simulink model "Earth_Pointing"  (R2020b)
settings: Solver=ode45  StartTime=0.0  StopTime=5829  RelTol=1e-5
values from neighbouring files (symbols this model uses):
  A = zeros(N_body+N_SP,1)    [main_detumbling.m]    (also in main_earthpointing.m; main_nocontrol.m)
  d = zeros(N_body+N_SP,3)    [main_detumbling.m]    (also in main_earthpointing.m; main_nocontrol.m)
  d_cg = [0.017 0 0]'    [main_detumbling.m]    (also in main_earthpointing.m; main_nocontrol.m)
  I = [Ix Iy Iz]    [main_detumbling.m]    (also in main_earthpointing.m; main_nocontrol.m)
  i = deg2rad(20)    [main_detumbling.m]    (also in main_earthpointing.m; main_nocontrol.m)
  IGRF_coefficients = [1 1 2 2 2 3 3 3 3 4 4 4 ... (832 elements, 104x8)]    [IGRF_coefficients.mat]
  kep = [a; e; i; OM; om; theta]    [main_detumbling.m]    (also in main_earthpointing.m; main_nocontrol.m)
  N = zeros(N_body+N_SP,3)    [main_detumbling.m]    (also in main_earthpointing.m; main_nocontrol.m)
  theta = 0    [PlotEarth.m]    (also in main_detumbling.m = deg2rad(0); main_earthpointing.m = deg2rad(0); main_nocontrol.m = deg2rad(0))
  w_0 = deg2rad([8 13 4])    [main_detumbling.m]    (also in main_earthpointing.m = deg2rad([0 0 0]); main_nocontrol.m)
undefined symbols (not defined in the file or in its folder): deg, IAU, s
libraries: aerolibtransform2 x1, aerolibconvert2 x1, dspmtrx3 x1
settings Model: SimulationMode=accelerator  Creator=GianMarco  LastModifiedBy=GianMarco

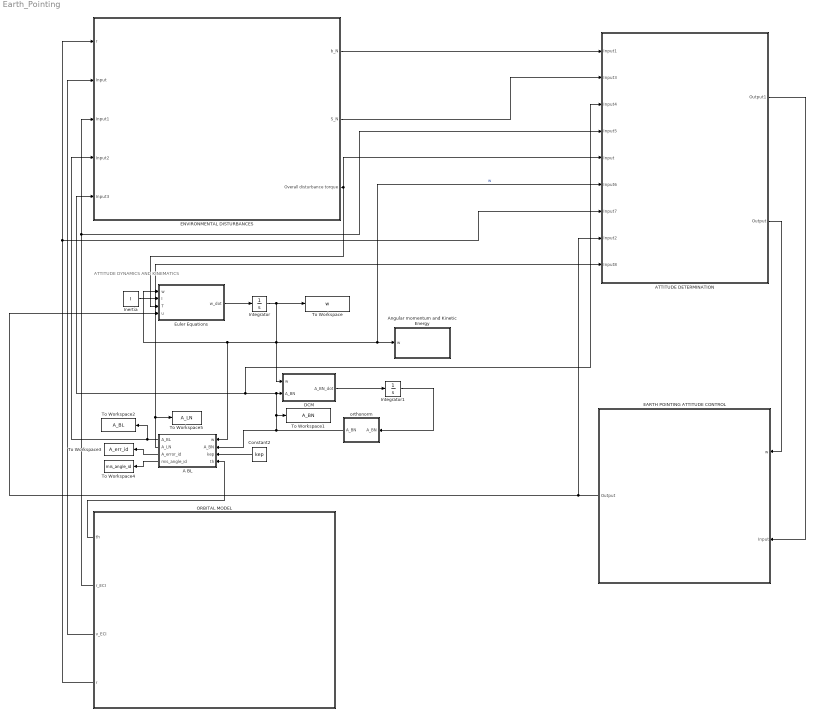
== system Earth_Pointing ==
  note: ATTITUDE DYNAMICS AND KINEMATICS
  A BL : MATLAB Function  TreatAsAtomicUnit=on
  ATTITUDE DETERMINATION : Subsystem
  Angular momentum and Kinetic Energy : Subsystem
  Constant2 : Constant  Value=kep
  DCM : MATLAB Function  TreatAsAtomicUnit=on
  EARTH POINTING ATTITUDE CONTROL : Subsystem  TreatAsAtomicUnit=on
  ENVIRONMENTAL DISTURBANCES : Subsystem
  Euler Equations : MATLAB Function  TreatAsAtomicUnit=on
  Inertia : Constant  Value=I
  Integrator : Integrator  InitialCondition=w_0
  Integrator1 : Integrator  InitialCondition="[-0.3579    0.7315    0.5804; 0.6621   -0.2396    0.7101; 0.6585    0.6384   -0.3986]"
  ORBITAL MODEL : Subsystem
  To Workspace : ToWorkspace  VariableName=w  SaveFormat=Timeseries  SampleTime=-1
  To Workspace1 : ToWorkspace  VariableName=A_BN  SampleTime=-1
  To Workspace2 : ToWorkspace  VariableName=A_BL  SampleTime=-1
  To Workspace3 : ToWorkspace  VariableName=A_err_id  SampleTime=-1
  To Workspace4 : ToWorkspace  VariableName=mis_angle_id  SampleTime=-1
  To Workspace5 : ToWorkspace  VariableName=A_LN  SampleTime=-1
  orthonorm : MATLAB Function  TreatAsAtomicUnit=on
  wires:
  Integrator/1 -> A BL/1(w), Euler Equations/1(w), DCM/1(w), Angular momentum and Kinetic Energy/1(w), ATTITUDE DETERMINATION/6(Input6), To Workspace/1  "w"
  Euler Equations/1(w_dot) -> Integrator/1
  Inertia/1 -> Euler Equations/2(I)
  DCM/1(A_BN_dot) -> Integrator1/1
  Integrator1/1 -> orthonorm/1("A_BN ")
  orthonorm/1(A_BN) -> ATTITUDE DETERMINATION/3(Input4), ENVIRONMENTAL DISTURBANCES/5(Input3), DCM/2(A_BN), To Workspace1/1, A BL/2(A_BN)
  Constant2/1 -> A BL/3(kep)
  ENVIRONMENTAL DISTURBANCES/3(Overall disturbance torque) -> ATTITUDE DETERMINATION/5(Input), Euler Equations/3(T)
  ORBITAL MODEL/2(r_ECI) -> ENVIRONMENTAL DISTURBANCES/3(Input1), ATTITUDE DETERMINATION/4(Input5)
  ORBITAL MODEL/3(v_ECI) -> ENVIRONMENTAL DISTURBANCES/2(Input)
  ORBITAL MODEL/1(th) -> A BL/4(th)
  ORBITAL MODEL/4(r) -> ENVIRONMENTAL DISTURBANCES/1(r), ATTITUDE DETERMINATION/7(Input7)
  A BL/1(A_BL) -> To Workspace2/1, ENVIRONMENTAL DISTURBANCES/4(Input2)
  ENVIRONMENTAL DISTURBANCES/2(S_N) -> ATTITUDE DETERMINATION/2(Input3)
  ENVIRONMENTAL DISTURBANCES/1(b_N) -> ATTITUDE DETERMINATION/1(Input1)
  ATTITUDE DETERMINATION/2(Output) -> EARTH POINTING ATTITUDE CONTROL/1(w)
  EARTH POINTING ATTITUDE CONTROL/1(Output) -> ATTITUDE DETERMINATION/8(Input2), Euler Equations/4(u)
  A BL/2(A_LN) -> To Workspace5/1, ATTITUDE DETERMINATION/9(Input8)
  ATTITUDE DETERMINATION/1(Output1) -> EARTH POINTING ATTITUDE CONTROL/2(Input)
  A BL/3(A_error_id) -> To Workspace3/1
  A BL/4(mis_angle_id) -> To Workspace4/1

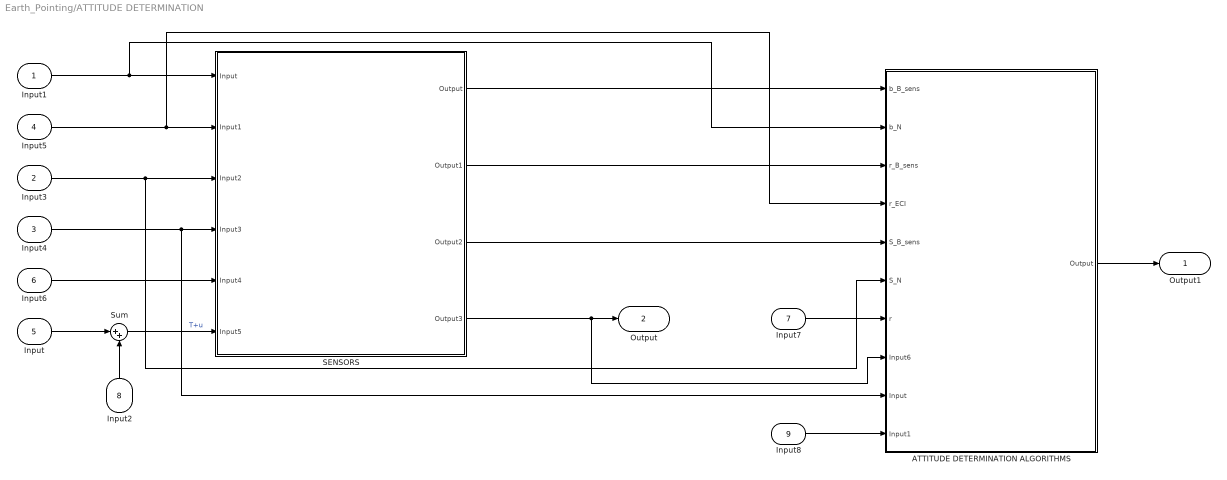
== system Earth_Pointing/ATTITUDE DETERMINATION ==
  Input1 : Inport
  Input3 : Inport  Port=2
  Input4 : Inport  Port=3
  Input5 : Inport  Port=4
  Input : Inport  Port=5
  Input6 : Inport  Port=6
  Input7 : Inport  Port=7
  Input2 : Inport  Port=8
  Input8 : Inport  Port=9
  ATTITUDE DETERMINATION ALGORITHMS : Subsystem
  SENSORS : Subsystem
  Sum : Sum  Inputs=|++
  Output1 : Outport
  Output : Outport  Port=2
  wires:
  Input7/1 -> ATTITUDE DETERMINATION ALGORITHMS/7(r)
  Input5/1 -> ATTITUDE DETERMINATION ALGORITHMS/4(r_ECI), SENSORS/2(Input1)
  Input1/1 -> ATTITUDE DETERMINATION ALGORITHMS/2(b_N), SENSORS/1(Input)
  Input4/1 -> ATTITUDE DETERMINATION ALGORITHMS/9(Input), SENSORS/4(Input3)
  Input3/1 -> ATTITUDE DETERMINATION ALGORITHMS/6(S_N), SENSORS/3(Input2)
  SENSORS/1(Output) -> ATTITUDE DETERMINATION ALGORITHMS/1(b_B_sens)
  SENSORS/2(Output1) -> ATTITUDE DETERMINATION ALGORITHMS/3(r_B_sens)
  SENSORS/3(Output2) -> ATTITUDE DETERMINATION ALGORITHMS/5(S_B_sens)
  Input6/1 -> SENSORS/5(Input4)
  SENSORS/4(Output3) -> Output/1, ATTITUDE DETERMINATION ALGORITHMS/8(Input6)
  Input2/1 -> Sum/2
  Input/1 -> Sum/1
  Sum/1 -> SENSORS/6(Input5)  "T+u"
  Input8/1 -> ATTITUDE DETERMINATION ALGORITHMS/10(Input1)
  ATTITUDE DETERMINATION ALGORITHMS/1(Output) -> Output1/1

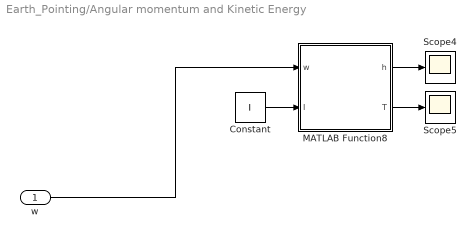
== system Earth_Pointing/Angular momentum and Kinetic Energy ==
  w : Inport
  Constant : Constant  Value=I
  MATLAB Function8 : MATLAB Function  TreatAsAtomicUnit=on
  Scope4 : Scope
  Scope5 : Scope
  wires:
  MATLAB Function8/1(h) -> Scope4/1
  w/1 -> MATLAB Function8/1(w)
  MATLAB Function8/2(T) -> Scope5/1
  Constant/1 -> MATLAB Function8/2(I)

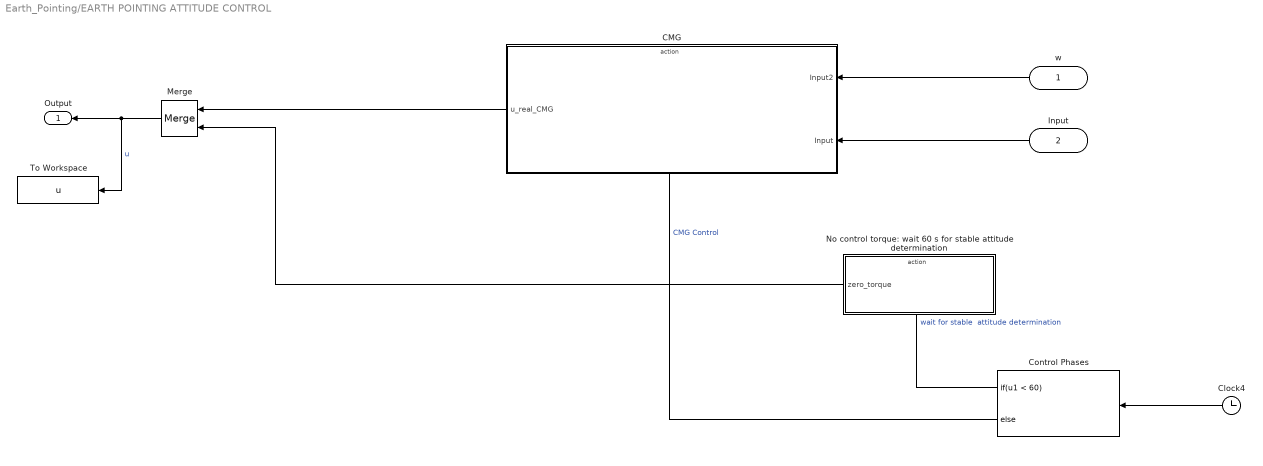
== system Earth_Pointing/EARTH POINTING ATTITUDE CONTROL ==
  w : Inport
  Input : Inport  Port=2
  CMG : Subsystem  TreatAsAtomicUnit=on
  Clock4 : Clock
  Control Phases : If  IfExpression=u1 < 60
  Merge : Merge
  No control torque: wait 60 s for stable attitude determination : Subsystem  TreatAsAtomicUnit=on
  To Workspace : ToWorkspace  VariableName=u  SampleTime=-1
  Output : Outport
  wires:
  Control Phases/1 -> No control torque: wait 60 s for stable attitude determination/Action  "wait for stable  attitude determination"
  No control torque: wait 60 s for stable attitude determination/1(zero_torque) -> Merge/2
  Merge/1 -> To Workspace/1, Output/1  "u"
  CMG/1(u_real_CMG) -> Merge/1
  Clock4/1 -> Control Phases/1
  Control Phases/2 -> CMG/Action  "CMG Control"
  w/1 -> CMG/1(Input2)
  Input/1 -> CMG/2(Input)

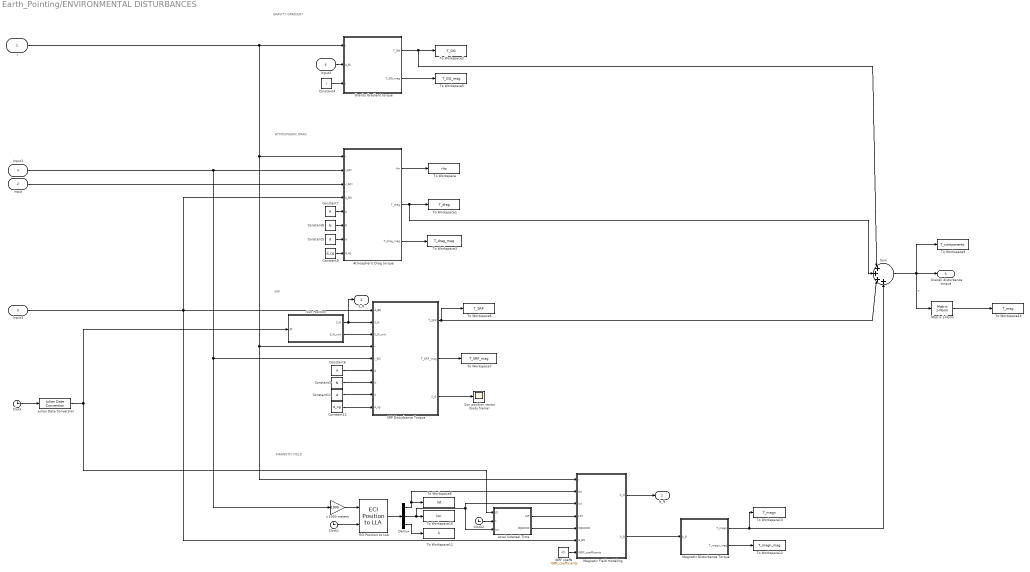
== system Earth_Pointing/ENVIRONMENTAL DISTURBANCES ==
  note: MAGNETIC FIELD
  note: ATMOSPHERIC DRAG
  note: GRAVITY GRADIENT
  note: SRP
  r : Inport
  Input : Inport  Port=2
  Input1 : Inport  Port=3
  Input2 : Inport  Port=4
  Input3 : Inport  Port=5
  Atmospheric Drag torque : MATLAB Function  TreatAsAtomicUnit=on
  Clock : Clock
  Clock1 : Clock
  Clock2 : Clock
  Constant11 : Constant  Value=d
  Constant12 : Constant  Value=d_cg
  Constant3 : Constant  Value=N
  Constant4 : Constant  Value=I
  Constant5 : Constant  Value=d
  Constant6 : Constant  Value=A
  Constant7 : Constant  Value=A
  Constant8 : Constant  Value=N
  Constant9 : Constant  Value=d_cg
  Demux : Demux  Outputs=3
  ECI Position to LLA : aerolibtransform2/ECI Position to LLA  red=IAU-2000/2006  year=2022  month=January  day=1  hour=12  min=0  sec=0  deltaT=Sec  errorflag=Error  extraparamflag=off  eunits=Metric (MKS)  earthmodel=WGS84  flat=1/298.257223563  eqradius=6378137
      settings: AttributesFormatString=%<red>  SourceProductBaseCode=AE
  Gravity Gradient torque : MATLAB Function  TreatAsAtomicUnit=on
  IGRF coeffs : Constant  Value=IGRF_coefficients
  Julian Date Conversion : aerolibconvert2/Julian Date Conversion  year=2022  month=January  day=1  hour=13  min=37  sec=9  modflag=off  deltaT=Sec  errorflag=Error
      settings: SourceProductBaseCode=AE
  Local Sidereal Time : MATLAB Function  TreatAsAtomicUnit=on
  Magnetic Disturbance Torque : MATLAB Function  TreatAsAtomicUnit=on
  Magnetic Field modeling : MATLAB Function  TreatAsAtomicUnit=on
  Matrix 1-Norm : dspmtrx3/Matrix  1-Norm  roundingMode=Floor  overflowMode=off  outputDataTypeStr=Inherit: Same as accumulator  outputMin=[]  outputMax=[]  outputLastDataTypeStr=Inherit: Same as accumulator
      settings: SourceProductBaseCode=DS
  SRP Disturbance Torque : MATLAB Function  TreatAsAtomicUnit=on
  Sum : Sum  Inputs=|++++
  Sun Position : MATLAB Function  TreatAsAtomicUnit=on
  Sun position vector (body frame) : Scope
  To Workspace : ToWorkspace  VariableName=rho  SampleTime=-1
  To Workspace1 : ToWorkspace  VariableName=T_drag  SampleTime=-1
  To Workspace10 : ToWorkspace  VariableName=lon  SampleTime=-1
  To Workspace11 : ToWorkspace  VariableName=h  SampleTime=-1
  To Workspace12 : ToWorkspace  VariableName=T_magn_mag  SampleTime=-1
  To Workspace13 : ToWorkspace  VariableName=T_magn  SampleTime=-1
  To Workspace14 : ToWorkspace  VariableName=T_mag  SampleTime=-1
  To Workspace2 : ToWorkspace  VariableName=T_GG  SampleTime=-1
  To Workspace3 : ToWorkspace  VariableName=T_drag_mag  SampleTime=-1
  To Workspace5 : ToWorkspace  VariableName=T_GG_mag  SampleTime=-1
  To Workspace6 : ToWorkspace  VariableName=T_SRP  SampleTime=-1
  To Workspace7 : ToWorkspace  VariableName=T_SRP_mag  SampleTime=-1
  To Workspace8 : ToWorkspace  VariableName=lat  SampleTime=-1
  To Workspace9 : ToWorkspace  VariableName=T_components  SampleTime=-1
  x 1000 meters : Gain  Gain=1000
  b_N : Outport
  S_N : Outport  Port=2
  Overall disturbance torque : Outport  Port=3
  wires:
  Constant4/1 -> Gravity Gradient torque/3(I)
  Gravity Gradient torque/1(T_GG) -> Sum/1, To Workspace2/1
  Gravity Gradient torque/2(T_GG_mag) -> To Workspace5/1
  Sun Position/1(S_N) -> SRP Disturbance Torque/2(S_N), S_N/1
  Julian Date Conversion/1 -> Local Sidereal Time/1(JD), Sun Position/1(JD)
  Clock/1 -> Julian Date Conversion/1
  Constant3/1 -> SRP Disturbance Torque/7(N)
  Constant11/1 -> SRP Disturbance Torque/8(d)
  SRP Disturbance Torque/3(S_B) -> Sun position vector (body frame)/1
  Sun Position/2(S_N_unit) -> SRP Disturbance Torque/3(S_N_unit)
  SRP Disturbance Torque/2(T_SRP_mag) -> To Workspace7/1
  Constant12/1 -> SRP Disturbance Torque/9(d_cg)
  SRP Disturbance Torque/1(T_SRP) -> To Workspace6/1, Sum/3
  Constant6/1 -> SRP Disturbance Torque/6(A)
  Magnetic Field modeling/1(b_N) -> b_N/1
  Magnetic Disturbance Torque/1(T_magn) -> To Workspace13/1, Sum/4
  Demux/2 -> To Workspace10/1, Local Sidereal Time/3(lon), Magnetic Field modeling/3(lon)
  x 1000 meters/1 -> ECI Position to LLA/1
  Demux/1 -> Magnetic Field modeling/2(lat), To Workspace8/1
  Clock2/1 -> Local Sidereal Time/2(t)
  Demux/3 -> To Workspace11/1
  IGRF coeffs/1 -> Magnetic Field modeling/7(IGRF_coefficients)
  Clock1/1 -> ECI Position to LLA/2
  Magnetic Field modeling/2(b_B) -> Magnetic Disturbance Torque/1(b_B)
  ECI Position to LLA/1 -> Demux/1
  Local Sidereal Time/1(LST) -> Magnetic Field modeling/4(LST)
  Local Sidereal Time/2(MJD2000) -> Magnetic Field modeling/5(MJD2000)
  Magnetic Disturbance Torque/2(T_magn_mag) -> To Workspace12/1
  Constant7/1 -> Atmospheric Drag torque/5(A)
  Constant8/1 -> Atmospheric Drag torque/6(N)
  Constant5/1 -> Atmospheric Drag torque/7(d)
  Constant9/1 -> Atmospheric Drag torque/8(d_cg)
  Input/1 -> Atmospheric Drag torque/3(v_ECI)
  Input1/1 -> x 1000 meters/1, SRP Disturbance Torque/5(r_ECI), Atmospheric Drag torque/2(r_ECI)
  r/1 -> Atmospheric Drag torque/1(r), SRP Disturbance Torque/4(r), Magnetic Field modeling/1(r), Gravity Gradient torque/1(r)
  Input2/1 -> Gravity Gradient torque/2(A_BL)
  Input3/1 -> Atmospheric Drag torque/4(A_BN), SRP Disturbance Torque/1(A_BN), Magnetic Field modeling/6(A_BN)
  Atmospheric Drag torque/1(rho) -> To Workspace/1
  Atmospheric Drag torque/3(T_drag_mag) -> To Workspace3/1
  Atmospheric Drag torque/2(T_drag) -> To Workspace1/1, Sum/2
  Sum/1 -> Matrix 1-Norm/1, Overall disturbance torque/1, To Workspace9/1  "T"
  Matrix 1-Norm/1 -> To Workspace14/1

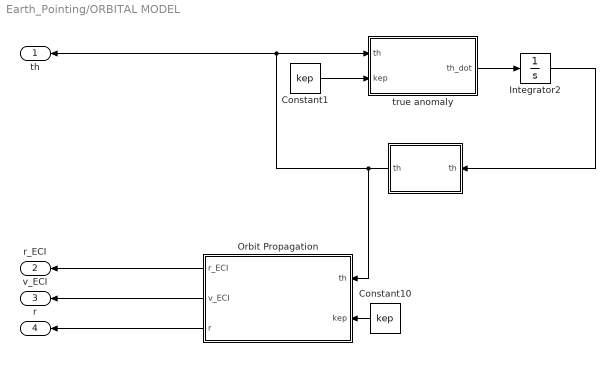
== system Earth_Pointing/ORBITAL MODEL ==
  " " : MATLAB Function  TreatAsAtomicUnit=on
  Constant1 : Constant  Value=kep
  Constant10 : Constant  Value=kep
  Integrator2 : Integrator  InitialCondition=theta
  Orbit Propagation : MATLAB Function  TreatAsAtomicUnit=on
  true anomaly : MATLAB Function  TreatAsAtomicUnit=on
  th : Outport
  r_ECI : Outport  Port=2
  v_ECI : Outport  Port=3
  r : Outport  Port=4
  wires:
  Orbit Propagation/3(r) -> r/1
  Orbit Propagation/2(v_ECI) -> v_ECI/1
  Constant1/1 -> true anomaly/2(kep)
  Integrator2/1 -> " "/1("th ")
  true anomaly/1(th_dot) -> Integrator2/1
  Orbit Propagation/1(r_ECI) -> r_ECI/1
  Constant10/1 -> Orbit Propagation/2(kep)
  " "/1(th) -> Orbit Propagation/1(th), th/1, true anomaly/1(th)

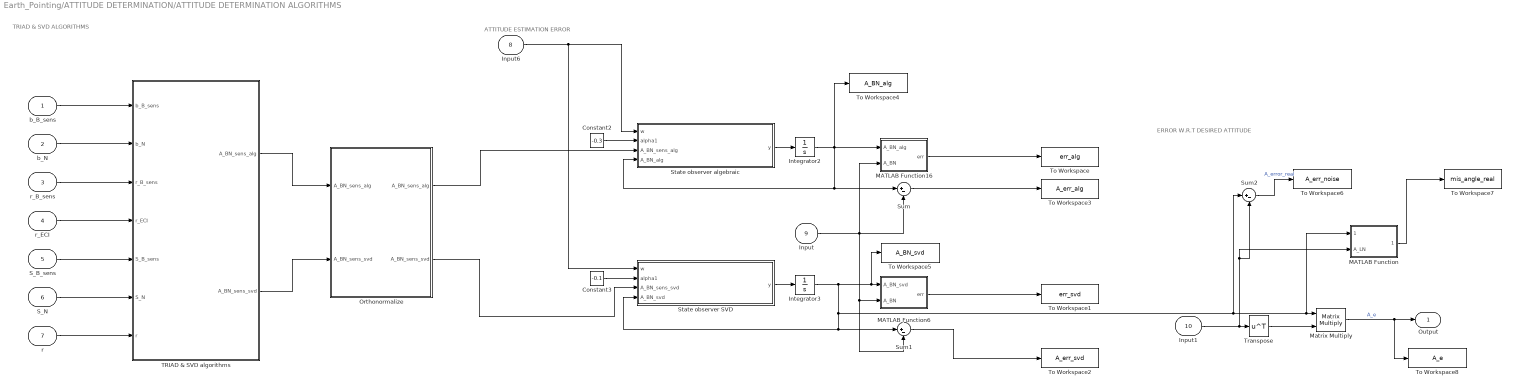
== system Earth_Pointing/ATTITUDE DETERMINATION/ATTITUDE DETERMINATION ALGORITHMS ==
  note: ERROR W.R.T DESIRED ATTITUDE
  note: ATTITUDE ESTIMATION ERROR
  note: TRIAD & SVD ALGORITHMS
  b_B_sens : Inport
  b_N : Inport  Port=2
  r_B_sens : Inport  Port=3
  r_ECI : Inport  Port=4
  S_B_sens : Inport  Port=5
  S_N : Inport  Port=6
  r : Inport  Port=7
  Input6 : Inport  Port=8
  Input : Inport  Port=9
  Input1 : Inport  Port=10
  Constant2 : Constant  Value=-0.3
  Constant3 : Constant  Value=-0.1
  Integrator2 : Integrator  InitialCondition=zeros(3,3)
  Integrator3 : Integrator  InitialCondition=zeros(3,3)
  MATLAB Function : MATLAB Function  TreatAsAtomicUnit=on
  MATLAB Function16 : MATLAB Function  TreatAsAtomicUnit=on
  MATLAB Function6 : MATLAB Function  TreatAsAtomicUnit=on
  Matrix Multiply : Product  Multiplication=Matrix(*)
  Orthonormalize : MATLAB Function  TreatAsAtomicUnit=on
  State observer SVD : MATLAB Function  TreatAsAtomicUnit=on
  State observer algebraic : MATLAB Function  TreatAsAtomicUnit=on
  Sum : Sum  Inputs=|+-
  Sum1 : Sum  Inputs=|+-
  Sum2 : Sum  Inputs=|+-
  TRIAD & SVD algorithms : MATLAB Function  TreatAsAtomicUnit=on
  To Workspace : ToWorkspace  VariableName=err_alg  SampleTime=-1
  To Workspace1 : ToWorkspace  VariableName=err_svd  SampleTime=-1
  To Workspace2 : ToWorkspace  VariableName=A_err_svd  SampleTime=-1
  To Workspace3 : ToWorkspace  VariableName=A_err_alg  SampleTime=-1
  To Workspace4 : ToWorkspace  VariableName=A_BN_alg  SampleTime=-1
  To Workspace5 : ToWorkspace  VariableName=A_BN_svd  SampleTime=-1
  To Workspace6 : ToWorkspace  VariableName=A_err_noise  SampleTime=-1
  To Workspace7 : ToWorkspace  VariableName=mis_angle_real  SampleTime=-1
  To Workspace8 : ToWorkspace  VariableName=A_e  SampleTime=-1
  Transpose : Math  Operator=transpose  SaturateOnIntegerOverflow=on
  Output : Outport
  wires:
  Constant2/1 -> State observer algebraic/2(alpha1)
  State observer SVD/1(y) -> Integrator3/1
  Orthonormalize/2(A_BN_sens_svd) -> State observer SVD/3(A_BN_sens_svd)
  TRIAD & SVD algorithms/2(A_BN_sens_svd) -> Orthonormalize/2("A_BN_sens_svd ")
  Sum1/1 -> To Workspace2/1
  Constant3/1 -> State observer SVD/2(alpha1)
  Integrator3/1 -> Sum1/1, State observer SVD/4(A_BN_svd), Sum2/1, MATLAB Function/1(A_BN_svd), Matrix Multiply/1, To Workspace5/1, MATLAB Function6/1(A_BN_svd)
  Sum/1 -> To Workspace3/1
  Orthonormalize/1(A_BN_sens_alg) -> State observer algebraic/3(A_BN_sens_alg)
  MATLAB Function16/1(err) -> To Workspace/1
  TRIAD & SVD algorithms/1(A_BN_sens_alg) -> Orthonormalize/1("A_BN_sens_alg ")
  MATLAB Function6/1(err) -> To Workspace1/1
  State observer algebraic/1(y) -> Integrator2/1
  Integrator2/1 -> Sum/1, State observer algebraic/4(A_BN_alg), MATLAB Function16/1(A_BN_alg), To Workspace4/1
  r/1 -> TRIAD & SVD algorithms/7(r)
  S_N/1 -> TRIAD & SVD algorithms/6(S_N)
  S_B_sens/1 -> TRIAD & SVD algorithms/5(S_B_sens)
  r_ECI/1 -> TRIAD & SVD algorithms/4(r_ECI)
  r_B_sens/1 -> TRIAD & SVD algorithms/3(r_B_sens)
  b_N/1 -> TRIAD & SVD algorithms/2(b_N)
  b_B_sens/1 -> TRIAD & SVD algorithms/1(b_B_sens)
  Input6/1 -> State observer SVD/1(w), State observer algebraic/1(w)
  Input/1 -> MATLAB Function16/2(A_BN), Sum/2, Sum1/2, MATLAB Function6/2(A_BN)
  Input1/1 -> Sum2/2, MATLAB Function/2(A_LN), Transpose/1
  Transpose/1 -> Matrix Multiply/2
  Matrix Multiply/1 -> To Workspace8/1, Output/1  "A_e"
  Sum2/1 -> To Workspace6/1  "A_error_real"
  MATLAB Function/1(mis_angle_real) -> To Workspace7/1

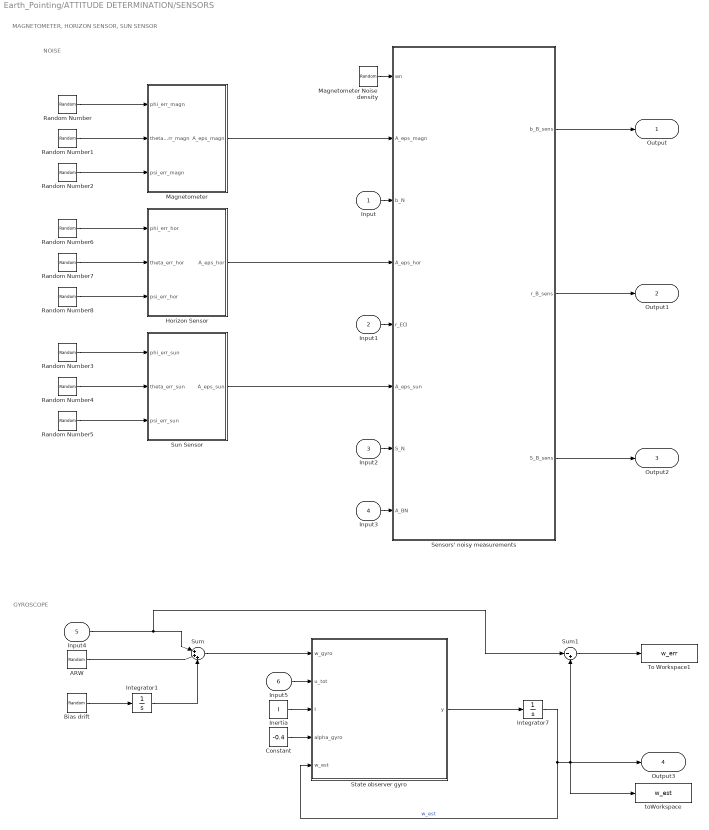
== system Earth_Pointing/ATTITUDE DETERMINATION/SENSORS ==
  note: MAGNETOMETER, HORIZON SENSOR, SUN SENSOR
  note: GYROSCOPE
  note: NOISE
  Input : Inport
  Input1 : Inport  Port=2
  Input2 : Inport  Port=3
  Input3 : Inport  Port=4
  Input4 : Inport  Port=5
  Input5 : Inport  Port=6
  ARW : RandomNumber  Variance=(deg2rad([0.15 0.15 0.15]/sqrt(3600))).^2 %[0.15 deg/s^.5]  SampleTime=1/250
  Bias drift : RandomNumber  Variance=(deg2rad([0.3 0.3 0.3]/3600)).^2  SampleTime=1/250
  Constant : Constant  Value=-0.4
  Horizon Sensor : MATLAB Function  TreatAsAtomicUnit=on
  Inertia : Constant  Value=I
  Integrator1 : Integrator  InitialCondition=[1/3600 1/3600 1/3600] % [deg/s], i.e. 1 deg/hour
  Integrator7 : Integrator  InitialCondition=[0 0 0]
  Magnetometer : MATLAB Function  TreatAsAtomicUnit=on
  Magnetometer Noise density : UniformRandomNumber  Minimum=1*1e-12  Maximum=16*1e-9  SampleTime=1/18
  Random Number : RandomNumber  Variance=deg2rad(1)  Seed=1  SampleTime=1/18
  Random Number1 : RandomNumber  Variance=deg2rad(1)  Seed=2  SampleTime=1/18
  Random Number2 : RandomNumber  Variance=deg2rad(1)  Seed=3  SampleTime=1/18
  Random Number3 : RandomNumber  Variance=deg2rad(1/100)  Seed=1  SampleTime=1/5
  Random Number4 : RandomNumber  Variance=deg2rad(1/100)  Seed=2  SampleTime=1/5
  Random Number5 : RandomNumber  Variance=deg2rad(1/100)  Seed=3  SampleTime=1/5
  Random Number6 : RandomNumber  Variance=deg2rad(1/16)  Seed=1  SampleTime=1
  Random Number7 : RandomNumber  Variance=deg2rad(1/16)  Seed=2  SampleTime=1
  Random Number8 : RandomNumber  Variance=deg2rad(1/16)  Seed=3  SampleTime=1
  Sensors' noisy measurements : MATLAB Function  TreatAsAtomicUnit=on
  State observer gyro : MATLAB Function  TreatAsAtomicUnit=on
  Sum : Sum  Inputs=|+++
  Sum1 : Sum  Inputs=|-+
  Sun Sensor : MATLAB Function  TreatAsAtomicUnit=on
  To Workspace1 : ToWorkspace  VariableName=w_err  SampleTime=-1
  toWorkspace : ToWorkspace  VariableName=w_est  SampleTime=-1
  Output : Outport
  Output1 : Outport  Port=2
  Output2 : Outport  Port=3
  Output3 : Outport  Port=4
  wires:
  Random Number2/1 -> Magnetometer/3(psi_err_magn)
  Random Number1/1 -> Magnetometer/2(theta_err_magn)
  Random Number/1 -> Magnetometer/1(phi_err_magn)
  Random Number4/1 -> Sun Sensor/2(theta_err_sun)
  Random Number5/1 -> Sun Sensor/3(psi_err_sun)
  Random Number6/1 -> Horizon Sensor/1(phi_err_hor)
  Random Number7/1 -> Horizon Sensor/2(theta_err_hor)
  Random Number8/1 -> Horizon Sensor/3(psi_err_hor)
  Random Number3/1 -> Sun Sensor/1(phi_err_sun)
  Magnetometer/1(A_eps_magn) -> Sensors' noisy measurements/2(A_eps_magn)
  Horizon Sensor/1(A_eps_hor) -> Sensors' noisy measurements/4(A_eps_hor)
  Sun Sensor/1(A_eps_sun) -> Sensors' noisy measurements/6(A_eps_sun)
  Input/1 -> Sensors' noisy measurements/3(b_N)
  Input1/1 -> Sensors' noisy measurements/5(r_ECI)
  Input2/1 -> Sensors' noisy measurements/7(S_N)
  Input3/1 -> Sensors' noisy measurements/8(A_BN)
  Sensors' noisy measurements/1(b_B_sens) -> Output/1
  Sensors' noisy measurements/2(r_B_sens) -> Output1/1
  Bias drift/1 -> Integrator1/1
  Input4/1 -> Sum1/1, Sum/1
  Integrator1/1 -> Sum/3
  Sum/1 -> State observer gyro/1(w_gyro)
  State observer gyro/1(y) -> Integrator7/1
  Integrator7/1 -> toWorkspace/1, Output3/1, Sum1/2, State observer gyro/5(w_est)  "w_est"
  Inertia/1 -> State observer gyro/3(I)
  Constant/1 -> State observer gyro/4(alpha_gyro)
  Input5/1 -> State observer gyro/2(u_tot)
  Sum1/1 -> To Workspace1/1
  Magnetometer Noise density/1 -> Sensors' noisy measurements/1(wn)
  Sensors' noisy measurements/3(S_B_sens) -> Output2/1
  ARW/1 -> Sum/2

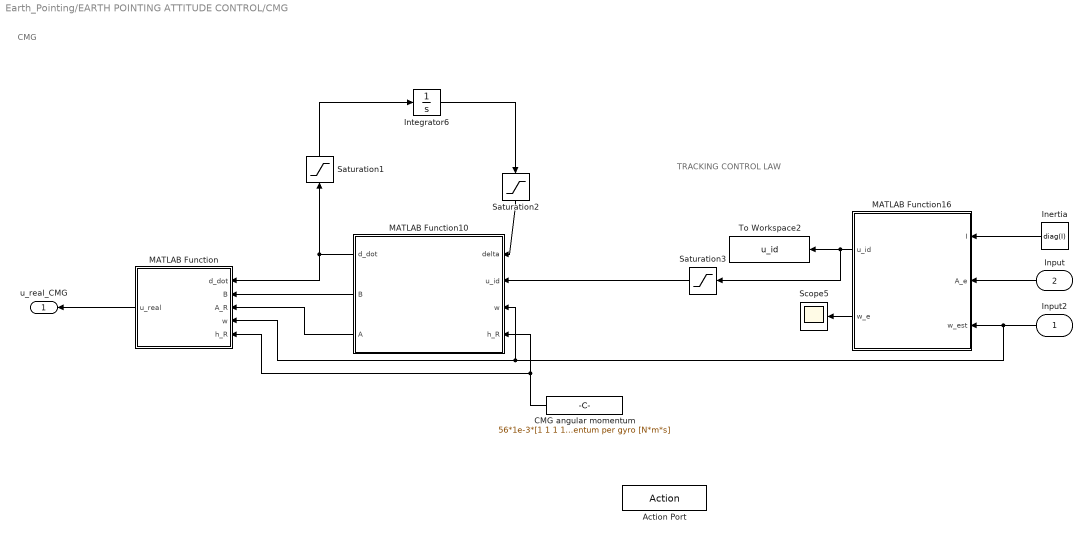
== system Earth_Pointing/EARTH POINTING ATTITUDE CONTROL/CMG ==
  note: CMG
  note: TRACKING CONTROL LAW
  Input2 : Inport
  Input : Inport  Port=2
  Action Port : ActionPort  ActionPortLabel=else
  CMG angular momentum : Constant  Value="56*1e-3*[1 1 1 1]'   % Angular momentum per gyro [N*m*s]"
  Inertia : Constant  Value=diag(I)
  Integrator6 : Integrator  InitialCondition=[0 0 0 0]'
  MATLAB Function : MATLAB Function  TreatAsAtomicUnit=on
  MATLAB Function10 : MATLAB Function  TreatAsAtomicUnit=on
  MATLAB Function16 : MATLAB Function  TreatAsAtomicUnit=on
  Saturation1 : Saturate  UpperLimit=deg2rad(20)  LowerLimit=-deg2rad(20)  ZeroCross=off
  Saturation2 : Saturate  UpperLimit=deg2rad(60)  LowerLimit=-deg2rad(60)  ZeroCross=off
  Saturation3 : Saturate  UpperLimit="0.112      % Max torque [N*m]"  LowerLimit="-0.112    % Max torque  [N*m]"
  Scope5 : Scope
  To Workspace2 : ToWorkspace  VariableName=u_id  SampleTime=-1
  u_real_CMG : Outport
  wires:
  MATLAB Function10/2(B) -> MATLAB Function/2(B)
  MATLAB Function/1(u_real) -> u_real_CMG/1
  CMG angular momentum/1 -> MATLAB Function10/4(h_R), MATLAB Function/5(h_R)
  Inertia/1 -> MATLAB Function16/1(I)
  MATLAB Function16/1(u_id) -> Saturation3/1, To Workspace2/1
  Saturation3/1 -> MATLAB Function10/2(u_id)
  MATLAB Function10/3(A) -> MATLAB Function/3(A_R)
  Saturation1/1 -> Integrator6/1
  MATLAB Function10/1(d_dot) -> MATLAB Function/1(d_dot), Saturation1/1
  Integrator6/1 -> Saturation2/1
  Input2/1 -> MATLAB Function16/3(w_est), MATLAB Function10/3(w), MATLAB Function/4(w)
  Saturation2/1 -> MATLAB Function10/1(delta)
  Input/1 -> MATLAB Function16/2(A_e)
  MATLAB Function16/2(w_e) -> Scope5/1

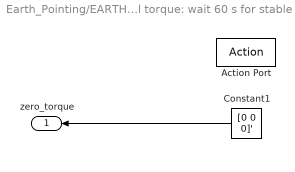
== system Earth_Pointing/EARTH POINTING ATTITUDE CONTROL/No control torque: wait 60 s for stable attitude determination ==
  Action Port : ActionPort  ActionPortLabel=if(u1 < 60)
  Constant1 : Constant  Value=[0 0 0]'
  zero_torque : Outport
  wires:
  Constant1/1 -> zero_torque/1

== matlab function Earth_Pointing/EARTH POINTING ATTITUDE CONTROL/CMG/MATLAB Function ==
  data: d_dot input; B input; A_R input; w input; h_R input; u_real output
function u_real  = cmg_torque(d_dot,B,A_R,w,h_R)

u_real = - cross(w,A_R*h_R) - B*d_dot;

end

== matlab function Earth_Pointing/ATTITUDE DETERMINATION/SENSORS/State observer gyro ==
  data: w_gyro input; u_tot input; I input; alpha_gyro input; w_est input; y output
function y = State_Observer(w_gyro, u_tot, I, alpha_gyro,w_est)


% Moments of Inertia [kg*m^2]
Ix = I(1);
Iy = I(2);
Iz = I(3);

Kx = (Iy-Iz)/Ix;
Ky = (Iz-Ix)/Iy;
Kz = (Ix-Iy)/Iz;


w_est_dot = zeros(3,1);
w_est_dot(1) = Kx * w_est(2)*w_est(3) + u_tot(1)/Ix + alpha_gyro*(w_est(1) - w_gyro(1));
w_est_dot(2) = Ky * w_est(1)*w_est(3) + u_tot(2)/Iy + alpha_gyro*(w_est(2) - w_gyro(2));
w_est_dot(3) = Kz * w_est(1)*w_est(2) + u_tot(3)/Iz + alpha_gyro*(w_est(3) - w_gyro(3));


y = w_est_dot;

== matlab function Earth_Pointing/EARTH POINTING ATTITUDE CONTROL/CMG/MATLAB Function10 ==
  data: delta input; u_id input; w input; d_dot output; h_R input; B output; A output
function [d_dot,B,A] = gimbal_angle_rate(delta,u_id,w,h_R)

% Gimbal moto angle 
b = deg2rad(54.73); 

% Tilt angles
d1 = delta(1);
d2 = delta(2);
d3 = delta(3);
d4 = delta(4);



A = [-cos(b)*sin(d1) -cos(d2)        cos(b)*sin(d3)   cos(d4);
       cos(d1)         -cos(b)*sin(d2) -cos(d3)         cos(b)*sin(d4);
       sin(b)*sin(d1)  sin(b)*sin(d2)  sin(b)*sin(d3)   sin(b)*sin(d4)];

h_r=h_R(1);

B = h_r * [-cos(b)*cos(d1) sin(d2)         cos(b)*cos(d3)  -sin(d4);
           sin(d1)         cos(b)*cos(d2)  -sin(d3)        -cos(b)*cos(d4);
           sin(b)*cos(d1)  sin(b)*cos(d2)  sin(b)*cos(d3)  sin(b)*cos(d4)];

d_dot = -pinv(B)*(u_id + cross(w,A*h_R));

== matlab function Earth_Pointing/ATTITUDE DETERMINATION/ATTITUDE DETERMINATION ALGORITHMS/MATLAB Function6 ==
  data: A_BN_svd input; err output; A_BN input
function err = fcn(A_BN_svd,A_BN)

% SVD Method Estimation error
err = abs(trace(A_BN_svd*A_BN' - eye(3)));

== matlab function Earth_Pointing/Angular momentum and Kinetic Energy/MATLAB Function8 ==
  data: w input; h output; T output; I input
function [h,T] = fcn(w,I)


Ix = I(1);
Iy = I(2);
Iz = I(3);

w_x=w(1);
w_y=w(2);
w_z=w(3); 

h=sqrt( (Ix*w_x)^2 + (Iy*w_y)^2 + (Iz*w_z)^2 );

T=Ix*w_x^2 + Iy*w_y^2 + Iz*w_z^2;

== matlab function Earth_Pointing/ENVIRONMENTAL DISTURBANCES/Gravity Gradient torque ==
  data: r input; T_GG output; A_BL input; I input; T_GG_mag output
function [T_GG,T_GG_mag]= GG(r,A_BL,I)

% Inertia moments of the 6U Cubesat with solar panels deployed [kg*m^2]
Ix=I(1);
Iy=I(2);
Iz=I(3);

%% GRAVITY GRADIENT TORQUE
% Gravitational constant and Earth's mass
G = 6.67408e-11; % [m^3*kg^-1*s^-2]
mt = 5.972e+24;  % [kg]

n = sqrt((3*G*mt)/(r*1e+3)^3);

% Direction cosines of the radial direction in principal axes
c = A_BL*[1 0 0]';

% GG disturbance torque [N*m]
T_GGx = (Iz-Iy)*n^2*c(3)*c(2);
T_GGy = (Ix-Iz)*n^2*c(1)*c(3);
T_GGz = (Iy-Ix)*n^2*c(2)*c(1);

T_GG = [T_GGx; T_GGy; T_GGz];

T_GG_mag = norm(T_GG);

== matlab function Earth_Pointing/ENVIRONMENTAL DISTURBANCES/Atmospheric Drag torque ==
  data: r input; r_ECI input; v_ECI input; A_BN input; A input; N input; d input; d_cg input; rho output; T_drag output; T_drag_mag output
function [rho,T_drag,T_drag_mag]  = Drag(r,r_ECI,v_ECI,A_BN,A,N,d,d_cg)

%% Atmospheric density exponential model

% Earth radius
R_E = 6378.137; % [km]

% Altitude
h = r - R_E; % [km]

H = 0;
h0 = 0;
rho_0 = 0; 

if h > 200 && h <= 250
    H = 37.105;
    h0 = 200;
    rho_0 = 2.789e-10;
elseif h > 250 && h <= 300
    H = 45.546;
    h0 = 250;
    rho_0 = 7.248e-11;
elseif h > 300 && h <= 350
    H = 53.628;
    h0 = 300;
    rho_0 = 2.418e-11;
elseif h > 350 && h <= 400
    H = 53.298;
    h0 = 350;
    rho_0 = 9.158e-12;
elseif h > 400 && h <= 450
    H = 58.515;
    h0 = 400;
    rho_0 = 3.725e-12;
elseif h > 450 && h <= 500
    H = 60.828;
    h0 = 450;
    rho_0 = 1.585e-12;
elseif h > 500 && h <= 600
    H = 63.822;
    h0 = 500;
    rho_0 = 6.967e-13;
elseif h > 600 && h <= 700
    H = 71.835;
    h0 = 600;
    rho_0 = 1.454e-13;
elseif h > 700 && h <= 800
    H = 88.667;
    h0 = 700;
    rho_0 = 3.614e-14;
elseif h > 800 && h <= 900
    H = 124.64;
    h0 = 800;
    rho_0 = 1.170e-14;
elseif h > 900 && h < 1000
    H = 181.05;
    h0 = 900;
    rho_0 = 5.245e-15;
elseif h > 1000 
    H = 268.0;
    h0 = 1000;
    rho_0 = 3.019e-15;
end

rho = rho_0*exp(-(h-h0)/H); % [kg/m^3]


%% Atmospheric Drag Torque

% Earth's angular rate and radius: 
w_E = 2*pi/(23*3600 + 56*60 + 4.09); % [rad/s]

% Relative atmosphere velocity with respect to the inertial frame
v_rel_N = (v_ECI + cross([0 0 w_E]', r_ECI))*1000; % [m/s]

% Relative atmosphere velocity expressed in body frame
v_rel_B = (A_BN*v_rel_N);  % [m/s]
v_rel_B_unit = (v_rel_B/norm(v_rel_B));

% Number of sufaces considered
N_body = 6;
N_SP = 4;

% Drag coefficient
C_D = 2.2;

% Initialize vector
T_drag = zeros(3,1);

for k = 1:N_body+N_SP
    
    n_k = N(k,:)';
    
    if dot(n_k,v_rel_B_unit) > 0
        d_k = (d(k,:) - d_cg')';
        F_k = - 0.5 * C_D * rho * norm(v_rel_B)^2 * dot(n_k,v_rel_B_unit) * A(k) * v_rel_B_unit;
        T_drag_k = cross(d_k, F_k);
    else
        T_drag_k = zeros(3,1);
    end
    
    T_drag = T_drag + T_drag_k;
    
    T_drag_mag = norm(T_drag);
end

== matlab function Earth_Pointing/ENVIRONMENTAL DISTURBANCES/SRP Disturbance Torque ==
  data: A_BN input; S_N input; S_N_unit input; T_SRP output; r input; r_ECI input; A input; N input; d input; d_cg input; T_SRP_mag output; S_B output
function [T_SRP, T_SRP_mag,S_B] = SRP(A_BN,S_N,S_N_unit,r,r_ECI,A,N,d,d_cg)

% Sun position vector with respect to body frame
S_B = A_BN*S_N;
S_B_norm = norm(S_B);
S_B_unit = S_B/S_B_norm;

% Earth radius [km]
R_E = 6378.137; 

% Shadow model
if dot(r_ECI,S_N_unit) < - sqrt(r^2 - R_E^2)
F  = 141.9; % [W/m^2]
else 
F = 1358 + 534.4 + 141.9; % [W/m^2] 
end

% Speed of light in vaccum [m/s]
c = 299792458; 

% Solar pressure
P = F/c;


% Number of surfaces considered
N_body = 6;
N_SP = 4;

% Specular and diffuse reflection coefficients
c_s_body = 0.5;     
c_d_body = 0.1;
c_s_SP = 0.8;
c_d_SP = 0.1;

% Compute SRP torque
T_SRP = zeros(3,1);

for k = 1:N_body+N_SP
    if k <= N_body
        c_s = c_s_body;     c_d = c_d_body;
    else
        c_s = c_s_SP;       c_d = c_d_SP;
    end
    
    n_k = N(k,:)';
    
    if dot(S_B_unit, n_k) > 0
        F_k = - P*A(k)*dot(S_B_unit,n_k) * ( (1-c_s)*S_B_unit + (2*c_s*dot(S_B_unit,n_k)+2/3*c_d)*n_k );
        d_k = (d(k,:) - d_cg')';
        T_SRP_k = cross(d_k, F_k);
    else
        T_SRP_k = zeros(3,1);
    end
    
    T_SRP = T_SRP + T_SRP_k;
    
        
end

T_SRP_mag = norm(T_SRP);

== matlab function Earth_Pointing/ENVIRONMENTAL DISTURBANCES/Sun Position ==
  data: S_N output; JD input; S_N_unit output
function [S_N,S_N_unit] = SunPosition(JD)

% From Markley, Crassidis: Fundamentals of Spacecraft Attitude
% Determination & Control (2014), pag. 420-422.

% Time T_0 in Julian centuries between the Julian day JD and J2000
T_0 = (JD - 2451545)/36525;

% Sun's Mean Longitude and Mean Anomaly [deg]
phi_sun = 280.460 + 36000.771*T_0;

M_sun = 357.5277233 + 35999.05034*T_0;

% Wrap to 360° 
if (phi_sun >= 360)
phi_sun = phi_sun - fix(phi_sun/360)*360; 
elseif (phi_sun < 0)
phi_sun = phi_sun - (fix(phi_sun/360) - 1)*360; 
end

if (M_sun >= 360)
M_sun = M_sun - fix(M_sun/360)*360; 
elseif (M_sun < 0)
M_sun = M_sun - (fix(M_sun/360) - 1)*360; 
end

% Ecliptic longitude 
phi_ecl = phi_sun + 1.914666471*sind(M_sun) + 0.019994643*sind(2*M_sun);

% Obliquity of the ecliptic
eps_ecl = 23.439291 - 0.0130042*T_0;

% Unit vector in the direction from Earth to Sun
S_N_unit = [cosd(phi_ecl); cosd(eps_ecl)*sind(phi_ecl); sind(eps_ecl)*sind(phi_ecl)];

% Distance between the Earth and the Sun [AU]
R_S = 1.000140612 - 0.016708617*cosd(M_sun) - 0.000139589*cosd(2*M_sun);

% Position vector from the Earth to the Sun 
S_N = R_S*S_N_unit; % [AU]

S_N = S_N*149597870.691; % [km]

== matlab function Earth_Pointing/ENVIRONMENTAL DISTURBANCES/Local Sidereal Time ==
  data: JD input; LST output; t input; lon input; MJD2000 output
function [LST,MJD2000] = LST(JD,t,lon)

% Adapted from: H.D. Curtis: Orbital Mechanics for Engineering Students
% (2014), pag.261. 

% Time T_0 in Julian centuries between the Julian day JD and J2000
T_0 = (JD - 2451545)/36525;

% Modified Julian Date
MJD2000 = JD - 2400000.5 - 51544.5;

% Greenwich sidereal time at 0 h UT
theta_G0 = 100.4606184 + 36000.77004*T_0 + 0.000387933*T_0^2 - 2.583e-8*T_0^3;

% Reduce theta_G0 so it lies in the range 0 - 360 degrees
if (theta_G0 >= 360)
theta_G0 = theta_G0 - fix(theta_G0/360)*360; 
elseif (theta_G0 < 0)
theta_G0 = theta_G0 - (fix(theta_G0/360) - 1)*360; 
end

% Universal Time (UT) in hours 
UT_0 = 12;
UT = UT_0 + t/3600;

% Greenwich sidereal time
theta_G = theta_G0 + 360.98564724*UT/24;

% Local sidereal time
LST = theta_G + lon;

% Reduce LST to the range 0 - 360 degrees:
LST = LST - 360*fix(LST/360);

== matlab function Earth_Pointing/ENVIRONMENTAL DISTURBANCES/Magnetic Field modeling ==
  data: r input; b_N output; lat input; lon input; LST input; MJD2000 input; A_BN input; b_B output; IGRF_coefficients input
function [b_N,b_B] = MagneticField(r,lat,lon,LST,MJD2000,A_BN,IGRF_coefficients)

% Geocentric radius in [m]
r = r*10^3;

% Compute colatitude and longitude in radians
colat=(90-lat)*pi/180;
lon = lon*pi/180;

% Reference radius used in IGRF [m]
R_E = 6371.2*10^3; 

% Read in the g and h Schmidt quasi-normalized coefficients from .mat file
gn = IGRF_coefficients(:,1);
gm = IGRF_coefficients(:,2);
gvali = IGRF_coefficients(:,3);
gsvi = IGRF_coefficients(:,4);
hn = IGRF_coefficients(:,5);
hm = IGRF_coefficients(:,6);
hvali = IGRF_coefficients(:,7);
hsvi = IGRF_coefficients(:,8);

% Set the IGRF order
N = 13;
g = zeros(N,N+1);
h = zeros(N,N+1);

for x=1:length(gn)
    g(gn(x),gm(x)+1) = gvali(x) + gsvi(x)*MJD2000/365;
    h(hn(x),hm(x)+1) = hvali(x) + hsvi(x)*MJD2000/365;
end

% Initialize the variables:
% B_r    B in the radial direction
% B_th   B in the theta direction
% B_phi  B in the phi direction
% P      Associated Legendre polynomial evaluated at cos(theta)
%        The nomenclature for the recursive values generally follows
%        the form P10 = P(n-1,m-0)
% dP     Partial derivative of P with respect to theta

B_r = 0; B_th = 0; B_phi = 0;
P11 = 1; P10 = P11;
dP11 = 0; dP10 = dP11;
P20 = 0; dP20 = 0;

% Compute the magnetic field strenght in local tangential coordinates with
% recursive formulas
for m=0:N
    for n=1:N
        if m<=n
            % Compute the Legendre polynomials and their derivatives
            if n == m
                P2 = sin(colat)*P11;
                dP2 = sin(colat)*dP11 + cos(colat)*P11;
                P11 = P2; P10 = P11; P20 = 0;
                dP11 = dP2; dP10 = dP11; dP20 = 0;
            elseif n == 1
                P2 = cos(colat)*P10;
                dP2 = cos(colat)*dP10 - sin(colat)*P10;
                P20 = P10; P10 = P2;
                dP20 = dP10; dP10 = dP2;
            else
                K = ((n-1)^2-m^2)/((2*n-1)*(2*n-3));
                P2 = cos(colat)*P10 - K*P20;
                dP2 = cos(colat)*dP10 - sin(colat)*P10 - K*dP20;
                P20 = P10; P10 = P2;
                dP20 = dP10; dP10 = dP2;
            end
            
            % Calculate B_r, B_th, and B_phi
            B_r = B_r + (R_E/r)^(n+2)*(n+1)*...
                ((g(n,m+1)*cos(m*lon) + h(n,m+1)*sin(m*lon))*P2);
            B_th = B_th + (R_E/r)^(n+2)*...
                ((g(n,m+1)*cos(m*lon) + h(n,m+1)*sin(m*lon))*dP2);
            B_phi = B_phi + (R_E/r)^(n+2)*...
                (m*(-g(n,m+1)*sin(m*lon) + h(n,m+1)*cos(m*lon))* P2);
        end
    end
end

B_th = -B_th;
B_phi = -B_phi/sin(colat);

% Convert latitude and LST from degrees to radians
lat = lat*pi/180;
LST = LST*pi/180;

% Convert B_r, B_th, B_phi from tangential spherical to ECI coordinates
B_x = (B_r*cos(lat)+B_th*sin(lat))*cos(LST) - B_phi*sin(LST);
B_y = (B_r*cos(lat)+B_th*sin(lat))*sin(LST) + B_phi*cos(LST);
B_z = (B_r*sin(lat)-B_th*cos(lat));

% Compute the Magnetic Field Vector in Tesla
b_N = [B_x; B_y; B_z]*1e-9;

b_B = A_BN*b_N;

== matlab function Earth_Pointing/ENVIRONMENTAL DISTURBANCES/Magnetic Disturbance Torque ==
  data: b_B input; T_magn output; T_magn_mag output
function [T_magn,T_magn_mag] = Magnetic(b_B)

% Residual magnetic induction due to currents in the satellite [N*m/T]
m = [0.1; 0.1; 0.1];

% Magnetic disturbance torque [N*m]
T_magn = cross(m,b_B);

T_magn_mag = norm(T_magn);

== matlab function Earth_Pointing/ATTITUDE DETERMINATION/SENSORS/Magnetometer ==
  data: phi_err_magn input; A_eps_magn output; theta_err_magn input; psi_err_magn input
function A_eps_magn = fcn(phi_err_magn,theta_err_magn,psi_err_magn)

cp=cos(phi_err_magn);
sp=sin(phi_err_magn);

ct=cos(theta_err_magn);
st=sin(theta_err_magn);

cs=cos(psi_err_magn);
ss=sin(psi_err_magn);

A_eps_magn=[cs*ct cs*st*sp+ss*cp -cs*st*cp+ss*sp; -ss*ct -ss*st*sp+cs*cp ss*st*cp+cs*sp; st -ct*sp ct*cp];

== matlab function Earth_Pointing/ATTITUDE DETERMINATION/SENSORS/Sun Sensor ==
  data: phi_err_sun input; A_eps_sun output; theta_err_sun input; psi_err_sun input
function A_eps_sun = fcn(phi_err_sun,theta_err_sun,psi_err_sun)

cp=cos(phi_err_sun);
sp=sin(phi_err_sun);

ct=cos(theta_err_sun);
st=sin(theta_err_sun);

cs=cos(psi_err_sun);
ss=sin(psi_err_sun);

A_eps_sun=[cs*ct cs*st*sp+ss*cp -cs*st*cp+ss*sp; -ss*ct -ss*st*sp+cs*cp ss*st*cp+cs*sp; st -ct*sp ct*cp];

== matlab function Earth_Pointing/ATTITUDE DETERMINATION/SENSORS/Horizon Sensor ==
  data: phi_err_hor input; A_eps_hor output; theta_err_hor input; psi_err_hor input
function A_eps_hor = fcn(phi_err_hor,theta_err_hor,psi_err_hor)

cp=cos(phi_err_hor);
sp=sin(phi_err_hor);

ct=cos(theta_err_hor);
st=sin(theta_err_hor);

cs=cos(psi_err_hor);
ss=sin(psi_err_hor);

A_eps_hor=[cs*ct cs*st*sp+ss*cp -cs*st*cp+ss*sp; -ss*ct -ss*st*sp+cs*cp ss*st*cp+cs*sp; st -ct*sp ct*cp];

== matlab function Earth_Pointing/ATTITUDE DETERMINATION/SENSORS/Sensors' noisy measurements ==
  data: wn input; A_eps_magn input; b_N input; A_eps_hor input; r_ECI input; A_eps_sun input; b_B_sens output; S_N input; r_B_sens output; S_B_sens output; A_BN input
function [b_B_sens,r_B_sens,S_B_sens] = measurements(wn,A_eps_magn,b_N,A_eps_hor,r_ECI,A_eps_sun,S_N,A_BN)

b_B_sens = A_eps_magn*A_BN*b_N + wn;
r_B_sens = A_eps_hor*A_BN*r_ECI;
S_B_sens = A_eps_sun*A_BN*S_N;

== matlab function Earth_Pointing/EARTH POINTING ATTITUDE CONTROL/CMG/MATLAB Function16 ==
  data: I input; u_id output; A_e input; w_est input; w_e output
function [u_id,w_e]= ideal_tracking(I,A_e,w_est)


u_id = zeros(3,1);

% Map the skew-symmetric matrix of the attitude error to its corresponding
% vector
skew_Sym = A_e' - A_e; 
% Map the corresponding vector
skew_Sym_invHat = [-skew_Sym(2,3) skew_Sym(1,3) -skew_Sym(1,2)]';

% Desired angular velocity (LVLH)
w_d = [0 0 sqrt(398600/7000^3)]';
w_d_dot = [0 0 0]';

w_e = w_est - A_e*w_d;

k1=0.05; 
k2=0.001;

u_id = -k1*w_e - k2*skew_Sym_invHat + cross(w_est,I*w_est) + I*(A_e*w_d_dot-cross(w_e,A_e*w_d));

end

== matlab function Earth_Pointing/ATTITUDE DETERMINATION/ATTITUDE DETERMINATION ALGORITHMS/TRIAD & SVD algorithms ==
  data: b_B_sens input; A_BN_sens_alg output; b_N input; r_B_sens input; r_ECI input; S_B_sens input; S_N input; A_BN_sens_svd output; r input
function [A_BN_sens_alg,A_BN_sens_svd]= TRIAD_SVD(b_B_sens,b_N,r_B_sens,r_ECI,S_B_sens,S_N,r)

% Normalize measurements to obtain unit vectors in body and inertial frames
b_B_sens_unit = b_B_sens/norm(b_B_sens);
b_N_unit = b_N/norm(b_N);

r_B_sens_unit = r_B_sens/norm(r_B_sens);
r_ECI_unit = r_ECI/norm(r_ECI);

S_B_sens_unit = S_B_sens/norm(S_B_sens);
S_N_unit = S_N/norm(S_N);

% Earth radius 
R_E = 6378.137; % [km]

%% ALGEBRAIC 

    p = b_B_sens_unit;
    q = r_B_sens_unit;
    
    a = b_N_unit;
    b = r_ECI_unit;
    
    s1 = p;
    s2 = cross(p,q) / norm(cross(p,q));
    s3 = cross(p,s2);

    v1 = a;
    v2 = cross(a,b) / norm(cross(a,b));
    v3 = cross(a,v2);

    S = [s1 s2 s3];
    V_triad = [v1 v2 v3];
    A_BN_sens_alg = S*V_triad';
    

%% SVD
% Accuracy of the sensors
acc_magn = 1;
acc_hor=1/4;
acc_sun = 1/8;

prec_magn = 1/acc_magn;
prec_hor = 1/acc_hor;
prec_sun = 1/acc_sun;

% If satellite is in shadow only 2 measurements are available:
if dot(r_ECI,S_N_unit) < - sqrt(r^2 - R_E^2)
    % Determine alpha coefficients
    alpha_magn = prec_magn / (prec_magn+prec_hor);
    alpha_hor =  prec_hor / (prec_magn+prec_hor);
    
    % Assemble B matrix
    B = alpha_magn*b_B_sens_unit*b_N_unit' + alpha_hor*r_B_sens_unit*r_ECI_unit';

else % 3 measurements are available
    % Determine alpha coefficients
    alpha_magn = prec_magn / (prec_magn+prec_sun+prec_hor);
    alpha_hor = prec_hor / (prec_magn+prec_sun+prec_hor);
    alpha_sun = prec_sun / (prec_magn+prec_sun+prec_hor);
    
    % Assemble B matrix
    B = alpha_magn*b_B_sens_unit*b_N_unit' + alpha_hor*r_B_sens_unit*r_ECI_unit'+ alpha_sun*S_B_sens_unit*S_N_unit';
end

% Perform Singular Value Decomposition
[U,~,V] = svd(B);
M = diag([1, 1, det(U)*det(V)]);
A_BN_sens_svd = U*M*V';

== matlab function Earth_Pointing/Euler Equations ==
  data: w input; I input; w_dot output; T input; u input
function w_dot = Euler_Equations(w,I,T,u)

% Inertia moments of the 6U Cubesat with solar panels deployed [kg*m^2]
Ix = I(1);
Iy = I(2);
Iz = I(3);

Kx=(Iy-Iz)/Ix;
Ky=(Iz-Ix)/Iy;
Kz=(Ix-Iy)/Iz;

% Euler Equations
w_dot = zeros(3,1);
w_dot(1)=Kx*w(2)*w(3) + (u(1)+T(1))/Ix;
w_dot(2)=Ky*w(1)*w(3) + (u(2)+T(2))/Iy;
w_dot(3)=Kz*w(1)*w(2) + (u(3)+T(3))/Iz;

== matlab function Earth_Pointing/ATTITUDE DETERMINATION/ATTITUDE DETERMINATION ALGORITHMS/Orthonormalize ==
  data: A_BN_sens_alg input; A_BN_sens_alg output; A_BN_sens_svd input; A_BN_sens_svd output
function [A_BN_sens_alg,A_BN_sens_svd] = orthonorm(A_BN_sens_alg,A_BN_sens_svd)

for k=1:3
A_BN_sens_alg=3/2 * A_BN_sens_alg - 1/2 * A_BN_sens_alg*A_BN_sens_alg'*A_BN_sens_alg;
A_BN_sens_svd=3/2 * A_BN_sens_svd - 1/2 * A_BN_sens_svd*A_BN_sens_svd'*A_BN_sens_svd;
end

== matlab function Earth_Pointing/ATTITUDE DETERMINATION/ATTITUDE DETERMINATION ALGORITHMS/State observer algebraic ==
  data: w input; alpha1 input; A_BN_sens_alg input; A_BN_alg input; y output
function y = State_Observer(w, alpha1,A_BN_sens_alg, A_BN_alg)


W = [0,    -w(3),  w(2);
     w(3),   0,   -w(1);
    -w(2),  w(1),   0];


A_BN_alg_dot = -W * A_BN_alg + alpha1*(A_BN_alg-A_BN_sens_alg);


y = A_BN_alg_dot;

== matlab function Earth_Pointing/ATTITUDE DETERMINATION/ATTITUDE DETERMINATION ALGORITHMS/State observer SVD ==
  data: w input; alpha1 input; A_BN_sens_svd input; A_BN_svd input; y output
function y = State_Observer(w, alpha1,A_BN_sens_svd, A_BN_svd)


W = [0,    -w(3),  w(2);
     w(3),   0,   -w(1);
    -w(2),  w(1),   0];


A_BN_svd_dot = -W * A_BN_svd + alpha1*(A_BN_svd-A_BN_sens_svd);


y = A_BN_svd_dot;

== matlab function Earth_Pointing/ATTITUDE DETERMINATION/ATTITUDE DETERMINATION ALGORITHMS/MATLAB Function16 ==
  data: A_BN_alg input; err output; A_BN input
function err = fcn(A_BN_alg,A_BN)

% Algebraic method estimation error
err = abs(trace(A_BN_alg*A_BN' - eye(3)));

== matlab function Earth_Pointing/ATTITUDE DETERMINATION/ATTITUDE DETERMINATION ALGORITHMS/MATLAB Function ==
  data: A_BN_svd input; mis_angle_real output; A_LN input
function mis_angle_real = fcn(A_BN_svd,A_LN)

mis_angle_real = rad2deg([(acos(dot(A_LN(1,:),A_BN_svd(1,:)))) (acos(dot(A_LN(2,:),A_BN_svd(2,:)))) (acos(dot(A_LN(3,:),A_BN_svd(3,:))))]);

== matlab function Earth_Pointing/DCM ==
  data: w input; A_BN_dot output; A_BN input
function A_BN_dot = DCM(w,A_BN)

W_cross = [0,    -w(3),  w(2);
           w(3),   0,   -w(1);
          -w(2),  w(1),   0];


A_BN_dot = -W_cross * A_BN;

== matlab function Earth_Pointing/orthonorm ==
  data: A_BN input; A_BN output
function A_BN = orthonorm(A_BN)

for k=1:3
A_BN=3/2 * A_BN - 1/2 * A_BN*A_BN'*A_BN;
end

== matlab function Earth_Pointing/ORBITAL MODEL/true anomaly ==
  data: th input; th_dot output; kep input
function th_dot = true_anomaly(th,kep)

% Semi-major axis [km] and eccentricity [-]
a = kep(1);
e = kep(2);

% Set Earth's standard gravitational parameter [km^3/s^2]
mu_E = 398600;  

% Orbital mean motion [rad/s]
n = sqrt(mu_E/a^3);  

% True anomaly derivative
th_dot = (n*(1+e*cos(th))^2)/((1-e^2)^(3/2));

== matlab function Earth_Pointing/A BL ==
  data: w input; A_BN input; kep input; th input; A_BL output; A_LN output; A_error_id output; mis_angle_id output
function [A_BL,A_LN,A_error_id,mis_angle_id] = fcn(w,A_BN,kep,th)

% Semi-major axis [km], Inclination [rad], RAAN [rad] and 
% Argument of perigee [rad]
a = kep(1);
i = kep(3);   
OM = kep(4);  
om = kep(5);  

% Rotation matrices
R3_omth = [cos(om+th) sin(om+th) 0; -sin(om+th) cos(om+th) 0; 0 0 1];
R1_i = [1 0 0; 0 cos(i) sin(i); 0 -sin(i) cos(i)];
R3_OM = [cos(OM) sin(OM) 0; -sin(OM) cos(OM) 0; 0 0 1];

% Rotation matrix Inertial frame --> LVLH (desired attitude)
A_LN = R3_omth*R1_i*R3_OM;

% Rotation matrix LVLH --> Body frame (attitude error)
A_BL = A_BN*A_LN';

A_error_id = A_BN-A_LN;


mis_angle_id = rad2deg([(acos(dot(A_LN(1,:),A_BN(1,:)))) (acos(dot(A_LN(2,:),A_BN(2,:)))) (acos(dot(A_LN(3,:),A_BN(3,:))))]);

== matlab function Earth_Pointing/ORBITAL MODEL/  ==
  data: th input; th output
function th = wrapto2pi(th)

% Wrap true anomaly between 0 and 2pi.

if th < 2*pi
    th=th;
else
    th=th-2*pi;
end
end

== matlab function Earth_Pointing/ORBITAL MODEL/Orbit Propagation ==
  data: th input; r_ECI output; kep input; v_ECI output; r output
function [r_ECI,v_ECI,r] = OrbitPropagation(th,kep)

% Orbital parameters
a = kep(1);
e = kep(2);
i = kep(3);
OM = kep(4);
om = kep(5);

% Semilatus rectum [km]
p = a*(1-e^2);

% Orbital radius [km]
r = p/(1+e*cos(th)); 

% Earth's standard gravitational parameter [km^3/s^2]
mu_E = 398600; 

% Rotation matrices: Earth-Centered Inertial --> Perifocal (ECI --> PF)
R_om = [cos(om)  sin(om)    0   ;
        -sin(om) cos(om)    0   ;
           0        0       1   ];
       
R_i  = [   1        0       0   ;
           0     cos(i)   sin(i);
           0    -sin(i)   cos(i)];
       
R_OM = [cos(OM)  sin(OM)    0   ;
        -sin(OM) cos(OM)    0   ;
           0        0       1   ];
    
R313 = R_om * R_i * R_OM; 

% Position and velocity vectors in perifocal coordinates
r_PF = r * [cos(th), sin(th), 0]';
v_PF = sqrt(mu_E/p) * [-sin(th), (e+cos(th)), 0]';

% PF --> ECI transformation
r_ECI = R313'* r_PF;
v_ECI = R313'* v_PF;
